simulink model "s_func_power"  (R2018b)
settings: Solver=VariableStepAuto  StartTime=0.0  StopTime=10.0  RelTol=1e-3
settings Model: Creator=student  LastModifiedBy=student

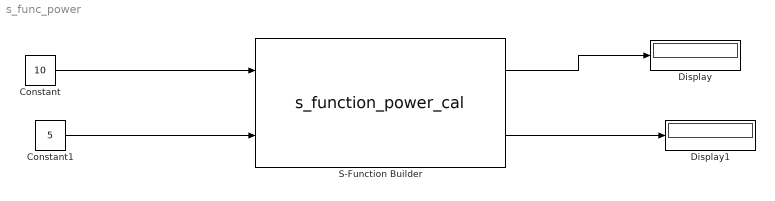
== system s_func_power ==
  Constant : Constant  Value=10
  Constant1 : Constant  Value=5
  Display : Display
  Display1 : Display
  S-Function Builder : S-Function  InitFcn=try, set_param(gcb,'FunctionName','s_function_power_cal'), end  FunctionName=s_function_power_cal  SFunctionModules=s_function_power_cal_wrapper  SFunctionDeploymentMode=off  EnableBusSupport=off  mask(S-Function Builder){}
      mask help: Simulink:masks:SFunctionBuilder_MD
      mask init:
      | val = [[.9  0.75 0.75 1 1 .9 .9 1]',[1 1 0.75 0.75 .9 .9 1 .9]'];try , sys = get_param(gcb,'SfunBuilderFcnName');if isempty(sys), sys = get_param(gcb,'FunctionName'); end,catch, sys = get_param(gcb,'FunctionName'); end
      settings: CopyFcn=set_param(gcbh,'LinkStatus','none')  PreSaveFcn=try, set_param(gcb,'FunctionName','s_function_power_cal'), end  OpenFcn=sfunctionwizard(gcbh)
      mask Display: plot(val(:,1),val(:,2)),disp(sys), port_label('input',1,'voltage'), port_label('input',2,'current'), port_label('output',1,'power'), port_label('output',2,'resistance')
  wires:
  Constant/1 -> S-Function Builder/1
  Constant1/1 -> S-Function Builder/2
  S-Function Builder/1 -> Display/1
  S-Function Builder/2 -> Display1/1
